simulink model "rtwdemo_bitfield"  (Simulink 7.1)
settings: Solver=FixedStepDiscrete  StartTime=0.0  StopTime=10.0  RelTol=1e-3
PostLoadFcn:
  | load bitfield_workspace.mat;
undefined symbols (not defined in the file or in its folder): p_1, p_2, p_3
settings Model: Creator=ajayaram  LastModifiedBy=ajayaram
settings SolverCC: AutoInsertRateTranBlk=on
settings DataIOCC: SaveOutput=off  SaveTime=off
settings OptimizationCC: InlineParams=on  InlineInvariantSignals=on  EnforceIntegerDowncast=off  StateBitsets=on  DataBitsets=on  UseTempVars=on  OptimizeModelRefInitCode=on  LifeSpan=1
settings RTWCC: SystemTargetFile=ert.tlc  GenCodeOnly=on  GenerateMakefile=off  TemplateMakefile=ert_default_tmf  Description=Real-Time Workshop Embedded Coder (no auto configuration)  GenerateReport=on  RTWVerbose=off  ProcessScript=ert_make_rtw_hook  IncludeHyperlinkInReport=on  LaunchReport=on
settings CodeAppCC: IgnoreCustomStorageClasses=off  CustomSymbolStrGlobalVar=rt$N$M  CustomSymbolStrType=$N$M  CustomSymbolStrFcn=$N$M$F  CustomSymbolStrMacro=$N$M
settings ERTTargetCC: GenerateSampleERTMain=on  SuppressErrorStatus=on  SupportAbsoluteTime=off  SupportNonFinite=off  SupportComplex=off  InlinedParameterPlacement=NonHierarchical  RootIOFormat=Structure reference  ERTCustomFileTemplate=example_file_process.tlc

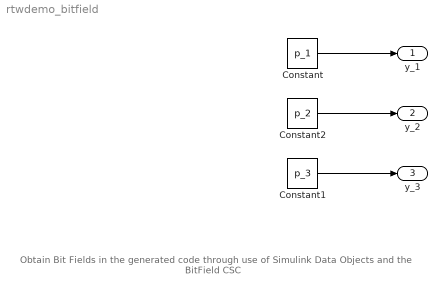
== system rtwdemo_bitfield ==
  note: Obtain Bit Fields in the generated code through use
      | of Simulink Data Objects and the BitField CSC
  Constant : Constant  Value=p_1  OutDataType=sfix(16)  OutScaling=2^0
  Constant1 : Constant  Value=p_3  OutDataType=sfix(16)  OutScaling=2^0
  Constant2 : Constant  Value=p_2  OutDataType=sfix(16)  OutScaling=2^0
  y_1 : Outport  OutDataType=sfix(16)  OutScaling=2^0
  y_2 : Outport  Port=2  OutDataType=sfix(16)  OutScaling=2^0
  y_3 : Outport  Port=3  OutDataType=sfix(16)  OutScaling=2^0
  wires:
  Constant/1 -> y_1/1
  Constant2/1 -> y_2/1
  Constant1/1 -> y_3/1
